simulink model "EarlyReturn2"  (R2020b)
settings: Solver=VariableStepAuto  StartTime=0.0  StopTime=10.0  RelTol=1e-3
settings Model: Creator=apple  LastModifiedBy=apple

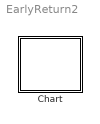
== system EarlyReturn2 ==
  Chart : Stateflow chart  TreatAsAtomicUnit=on

== stateflow chart EarlyReturn2/Chart ==
  state A
    en: fprintf("en_A")
    ex: fprintf("ex_A")
    state A1
      en: fprintf("en_A1")
      ex: fprintf("ex_A1")
    state A2
      en: fprintf("en_A2")
      ex: fprintf("ex_A2")
    (default) -> A1
    A1 -> A2 : {fprintf("E");E}/{fprintf("ta")}
  state B
    en: fprintf("en_B")
    ex: fprintf("ex_B")
  (default) -> A
  A -> B : E
  events: E local FUNCTION_CALL_EVENT
